simulink model "tp1ej2pD"  (R2024a)
settings: Solver=VariableStepAuto  StartTime=0.0  StopTime=60e-3  MaxStep=5e-6  RelTol=1e-3
undefined symbols (not defined in the file): b, J, Kb, Kt, L, R, Tp
settings Model: Creator=fab  LastModifiedBy=fab

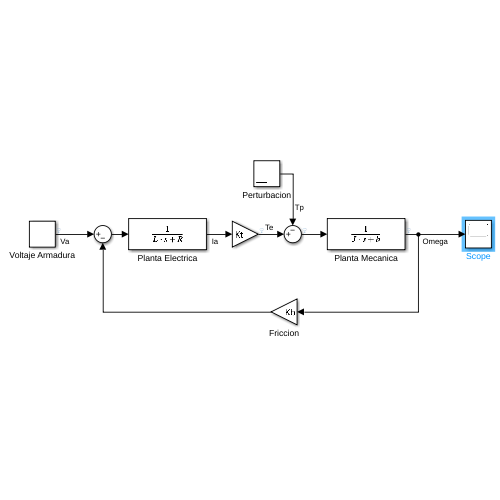
[thumbnail: Simulink's stored preview of the top-level diagram]
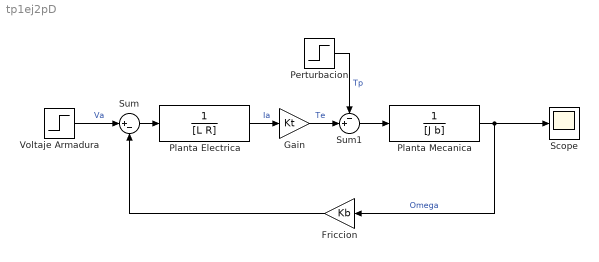
== system tp1ej2pD ==
  Friccion : Gain  Gain=Kb
  Gain : Gain  Gain=Kt
  Perturbacion : Step  Time=30e-3  After=Tp  SampleTime=0
  Planta Electrica : TransferFcn  Denominator=[L R]
  Planta Mecanica : TransferFcn  Denominator=[J b]
  Scope : Scope
  Sum : Sum  Inputs=|+-
  Sum1 : Sum  Inputs=-+|
  Voltaje Armadura : Step  Time=0  After=60  SampleTime=0
  wires:
  Voltaje Armadura/1 -> Sum/1  "Va"
  Friccion/1 -> Sum/2
  Gain/1 -> Sum1/2  "Te"
  Sum/1 -> Planta Electrica/1
  Planta Mecanica/1 -> Scope/1, Friccion/1  "Omega"
  Planta Electrica/1 -> Gain/1  "Ia"
  Sum1/1 -> Planta Mecanica/1
  Perturbacion/1 -> Sum1/1  "Tp"
